simulink library "csu_snm_sensonor_noise_model_lib"  (R2014b)
settings: Solver=ode45  SolverMode=SingleTasking  StartTime=0.0  StopTime=10.0  RelTol=1e-3
values from neighbouring files (symbols this model uses):
  mnm_dt = sim_time_step_size    [csu_mnm_mems_noise_model_init.m]
undefined symbols (not defined in the file or in its folder): sim_time_step_size, snm_accel_bias_v, snm_accel_noise_on, snm_accel_noise_seed_v, snm_accel_noise_v, snm_accel_range, snm_accel_SF, snm_correlation_time, snm_dt, snm_gyro_bias_v, snm_gyro_g_sensitive, snm_gyro_noise_on, snm_gyro_noise_seed_v, snm_gyro_noise_v, snm_gyro_range, snm_gyro_SF, snm_gyro_vibe_sensitive, snm_thrust_accel_bias, snm_thrust_accel_noise_factor, snm_thrust_gyro_noise_factor
libraries: util_common_lib x3, simulink x1, util_info_lib x1
settings Model: Creator=hcannon  LastModifiedBy=mstewart

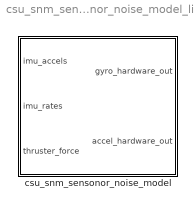
== system csu_snm_sensonor_noise_model_lib ==
  csu_snm_sensonor_noise_model : Subsystem

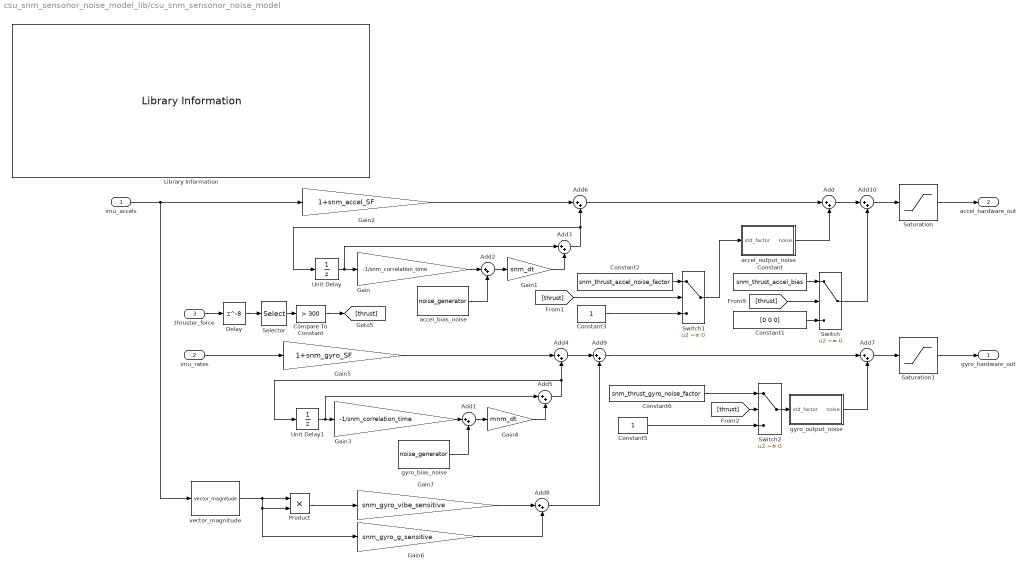
== system csu_snm_sensonor_noise_model_lib/csu_snm_sensonor_noise_model ==
  imu_accels : Inport
  imu_rates : Inport  Port=2
  thruster_force : Inport  Port=3
  Add{,1..10} (11 alike) : Sum  Inputs=|++
  Compare To Constant : simulink/Logic and Bit Operations/Compare To Constant  relop=>  const=300  OutDataTypeStr=boolean
  Constant : Constant  Value=snm_thrust_accel_bias  OutDataTypeStr=double
  Constant1 : Constant  Value=[0 0 0]  OutDataTypeStr=double
  Constant2 : Constant  Value=snm_thrust_accel_noise_factor  OutDataTypeStr=double
  Constant3 : Constant  OutDataTypeStr=double
  Constant5 : Constant  OutDataTypeStr=double
  Constant6 : Constant  Value=snm_thrust_gyro_noise_factor  OutDataTypeStr=double
  Delay : Delay  DelayLength=8  InitialCondition=0
  Gain : Gain  Gain=-1/snm_correlation_time
  Gain1 : Gain  Gain=snm_dt
  Gain2 : Gain  Gain=1+snm_accel_SF
  Gain3 : Gain  Gain=-1/snm_correlation_time
  Gain4 : Gain  Gain=mnm_dt
  Gain5 : Gain  Gain=1+snm_gyro_SF
  Gain6 : Gain  Gain=snm_gyro_g_sensitive
  Gain7 : Gain  Gain=snm_gyro_vibe_sensitive
  Library Information : util_info_lib/Library Information  owner='NONE'
  Product : Product  RndMeth=Zero
  Saturation : Saturate  UpperLimit=snm_accel_range  LowerLimit=-snm_accel_range
  Saturation1 : Saturate  UpperLimit=snm_gyro_range  LowerLimit=-snm_gyro_range
  Selector : Selector  InputPortWidth=3  Indices=[3]
  Switch : Switch  Criteria=u2 ~= 0
  Switch1 : Switch  Criteria=u2 ~= 0
  Switch2 : Switch  Criteria=u2 ~= 0
  Unit Delay : UnitDelay  SampleTime=-1
  Unit Delay1 : UnitDelay  SampleTime=-1
  accel_bias_noise : util_common_lib/noise_generator  std_dev=snm_accel_bias_noise_v  bias=snm_accel_bias_bias_v  seed=snm_accel_bias_seed_v  on=snm_accel_noise_on  sample_time=sim_time_step_size
  accel_output_noise : Subsystem
  gyro_bias_noise : util_common_lib/noise_generator  std_dev=snm_gyro_bias_noise_v  bias=snm_gyro_bias_bias_v  seed=snm_gyro_bias_seed_v  on=snm_gyro_noise_on  sample_time=sim_time_step_size
  gyro_output_noise : Subsystem
  vector_magnitude : util_common_lib/vector_magnitude  SystemSampleTime=-1
  gyro_hardware_out : Outport
  accel_hardware_out : Outport  Port=2
  wires:
  Delay/1 -> Selector/1
  Add7/1 -> Saturation1/1
  gyro_bias_noise/1 -> Add1/2
  Gain3/1 -> Add1/1
  imu_rates/1 -> Gain5/1
  Add5/1 -> Unit Delay1/1, Add4/2
  Unit Delay1/1 -> Add5/1, Gain3/1
  Gain4/1 -> Add5/2
  Add1/1 -> Gain4/1
  accel_bias_noise/1 -> Add2/2
  Gain/1 -> Add2/1
  imu_accels/1 -> Gain2/1, vector_magnitude/1
  Add3/1 -> Unit Delay/1, Add6/2
  Unit Delay/1 -> Add3/1, Gain/1
  Gain1/1 -> Add3/2
  Add2/1 -> Gain1/1
  Saturation1/1 -> gyro_hardware_out/1
  Gain5/1 -> Add4/1
  Gain2/1 -> Add6/1
  Add6/1 -> Add/1
  vector_magnitude/1 -> Product/1, Gain6/1, Product/2
  Product/1 -> Gain7/1
  Gain7/1 -> Add8/1
  Gain6/1 -> Add8/2
  Add4/1 -> Add9/1
  Add9/1 -> Add7/1
  Add8/1 -> Add9/2
  Add10/1 -> Saturation/1
  Saturation/1 -> accel_hardware_out/1
  [thrust] -> Switch/2
  Constant/1 -> Switch/1
  Constant1/1 -> Switch/3
  Add/1 -> Add10/1
  Switch/1 -> Add10/2
  thruster_force/1 -> Delay/1
  Compare To Constant/1 -> [thrust]
  [thrust] -> Switch1/2
  accel_output_noise/1(noise) -> Add/2
  Constant2/1 -> Switch1/1
  Constant3/1 -> Switch1/3
  [thrust] -> Switch2/2
  Constant6/1 -> Switch2/1
  Constant5/1 -> Switch2/3
  gyro_output_noise/1(noise) -> Add7/2
  Switch2/1 -> gyro_output_noise/1(std_factor)
  Selector/1 -> Compare To Constant/1
  Switch1/1 -> accel_output_noise/1(std_factor)

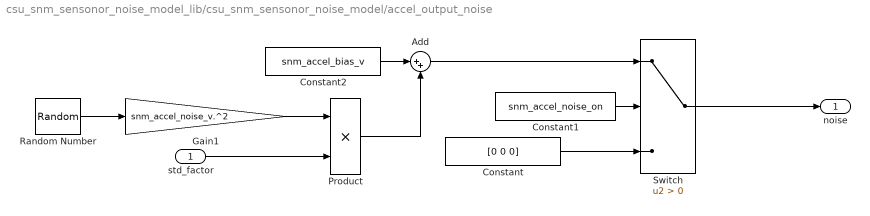
== system csu_snm_sensonor_noise_model_lib/csu_snm_sensonor_noise_model/accel_output_noise ==
  std_factor : Inport
  Add : Sum  Inputs=|++
  Constant : Constant  Value=[0 0 0]
  Constant1 : Constant  Value=snm_accel_noise_on
  Constant2 : Constant  Value=snm_accel_bias_v
  Gain1 : Gain  Gain=snm_accel_noise_v.^2
  Product : Product
  Random Number : RandomNumber  Mean=[0 0 0]  Variance=[1 1 1]  Seed=snm_accel_noise_seed_v  SampleTime=sim_time_step_size
  Switch : Switch  Criteria=u2 > Threshold
  noise : Outport
  wires:
  Switch/1 -> noise/1
  Constant/1 -> Switch/3
  Constant1/1 -> Switch/2
  Random Number/1 -> Gain1/1
  Product/1 -> Add/2
  Constant2/1 -> Add/1
  Add/1 -> Switch/1
  Gain1/1 -> Product/1
  std_factor/1 -> Product/2

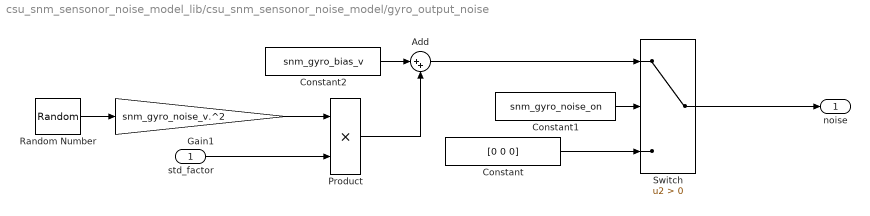
== system csu_snm_sensonor_noise_model_lib/csu_snm_sensonor_noise_model/gyro_output_noise ==
  std_factor : Inport
  Add : Sum  Inputs=|++
  Constant : Constant  Value=[0 0 0]
  Constant1 : Constant  Value=snm_gyro_noise_on
  Constant2 : Constant  Value=snm_gyro_bias_v
  Gain1 : Gain  Gain=snm_gyro_noise_v.^2
  Product : Product
  Random Number : RandomNumber  Mean=[0 0 0]  Variance=[1 1 1]  Seed=snm_gyro_noise_seed_v  SampleTime=sim_time_step_size
  Switch : Switch  Criteria=u2 > Threshold
  noise : Outport
  wires:
  Switch/1 -> noise/1
  Constant/1 -> Switch/3
  Constant1/1 -> Switch/2
  Random Number/1 -> Gain1/1
  Product/1 -> Add/2
  Constant2/1 -> Add/1
  Add/1 -> Switch/1
  Gain1/1 -> Product/1
  std_factor/1 -> Product/2
